simulink model "FOC_CHBI"  (R2025a)
settings: Solver=VariableStepAuto  StartTime=0.0  StopTime=6.5  RelTol=1e-3
InitFcn:
  | %% KHOI THONG SO DONG CO
  | U_nom=6000;%6600;           %dien ap dinh muc dong co
  | H=0.96;%0.9387;             %hieu suat dong co
  | Pn=1e6;%1750e3;         %Cong suat dinh muc dong co
  | cosphi=0.85;%0.9297;        %He so cong suat
  | Sn=Pn/cosphi;       %Cong suat toan phan
  | J=27.9;%34.8;                %Moment quan tinh
  | pc=2;%2;               %So cap cuc
  | fn=50;              %Tan so luoi
  | n=1490;%1486;             %Toc do dinh muc 2880
  | Mdm=6153;%(9.55*Pn*H)/n;  %Moment dinh muc
  | In=117;%Pn/(U_nom*H*cosphi*sqrt(3))   ;
  | Isd=sqrt(2)*In*sqrt(1-cosphi);
  | Isq=sqrt(2*In^2-Isd^2);
  | wrn=2*pi*(fn-(pc*n/60));               %Toc do truotdinh muc
  | Tr=Isq/(wrn*Isd) ;                   %Tinh 'Tr'trong cac cong thuc
  | %Xo=(sqrt(1-cosphi^2)-cosphi*Isd/Isq)*(Un*sqrt(2)/(sqrt(3)*In));
  | Xo=(sqrt(1-cosphi^2)-cosphi*Isd/Isq)*(U_nom/(sqrt(3)*In));
  | Xh=sqrt(2/3)*(U_nom/Isd) - Xo;
  | Rs=(wrn*Isd*Xh)/(2*pi*fn*Isq);
  | Rr=Rs;
  | o=Xo/Xh;
  | Ts=Xh/(2*pi*fn*Rs);
  | Tos=o*Ts;
  | Lr=Tr*Rr;
  | Lor=o*Lr;
  | Ls=Ts*Rs;
  | Los=o*Ls;
  | Lm=sqrt((1-o)*Ls*Lr);
  | %tham so dong co 2850e3Kw
  | %Rs=0.05;
  | %Rr = 0.062;
  | %Los = 0.957/(100*pi);
  | %Lor = 2.237/(100*pi);
  | %Lm = 34.826/(100*pi);
  | %Ts = (Lm +Los)/Rs;
  | %Tr = (Lm+Lor)/Rr;
  | %Lr = Lm + Lor;
  | %Ls = Lm + Los;
  | Udc = 1.1*6000/(0.612*12);%6600/(0.612*12);
  | Rt =18*Udc*Udc/1e6; %18*Udc*Udc/2010.6e3;
  | C_f = 5/(6*100*pi*Rt*0.001);
  | %Fan and Pumb Load Coeficient
  | TL0 = (2.0/100)*Mdm; %(2.0/100)*TN;
  | Omega_rated = n/9.55; %nN/9.55; %rad/s
  | LoadGain = (Mdm - TL0)/(Omega_rated*Omega_rated);
  | fs=5000;
  | %% THAM SO CAC BO DIEU KHIEN
  | %---------------- control volocity
  | epxilon = 0.7;
  | wn = 40;
  |      %P_w = (2*epxilon*wn*J)/pc;
  |     %I_w = wn*wn*J/pc;
  |  P_w = 60;%5;%15;%9;%12;%10;%(2*epxilon*wn*J)/pc
  |  I_w = 80;%150;%80;%100;%40;%50;%wn*wn*J/pc
  | %---------------- control current
  |     %P_id = Rs*Tos*fs/5;
  |     % I_id = Rs*Tos*fs/5/Tos;
  |      %P_iq = P_id;
  |      %I_iq = I_id;
  | ... (+9 lines)
StopFcn:
  | figure(1);
  | subplot(1,1,1); hold on; grid on;
  | plot(phi_ref.time, phi_ref.signals.values,'r--', 'Linewidth',1.5);
  | plot(phi.time, phi.signals.values,'b', 'Linewidth',1.5);
  | legend('phi*-rd','phi-rd');
  | title('Từ thông');
  | xlabel('Thời gian (s)'); ylabel('Wb');
  | 
  | 
  | figure(2);
  | subplot(2,1,1); hold on; grid on;
  | plot(torque.time, torque.signals.values,'r','Linewidth',1.5);
  | legend('Te');
  | title('Mô-men');
  | xlabel('Thời gian (s)'); ylabel('Nm');
  | 
  | subplot(2,1,2); hold on; grid on;
  | plot(speed_ref.time, speed_ref.signals.values,'r--','Linewidth',1.5);
  | plot(speed.time, speed.signals.values,'b','Linewidth',1.5);
  | legend('Tốc độ đặt','Tốc độ thực');
  | title('Tốc độ');
  | xlabel('Thời gian (s)'); ylabel('RPM');
  | 
  | figure(3)
  | 
  | subplot(2,1,1); hold on; grid on;
  | plot(isd_ref.time, isd_ref.signals.values,'r','Linewidth',1.5);
  | plot(isd.time, isd.signals.values,'b','Linewidth',1.5);
  | legend('isd*','isd');
  | title('Dòng điện isd');
  | xlabel('Thời gian (s)'); ylabel('A');
  | 
  | subplot(2,1,2); hold on; grid on;
  | plot(isq_ref.time, isq_ref.signals.values,'r','Linewidth',1.5);
  | plot(isq.time, isq.signals.values,'b','Linewidth',1.5);
  | legend('isq*','isq');
  | title('Dòng điện isq');
  | xlabel('Thời gian (s)'); ylabel('A');
  | 
  | figure(4)
  | 
  | subplot(2,1,1); hold on; grid on;
  | plot(va.time, va.signals.values,'b','Linewidth',1.5);
  | plot(vb.time, vb.signals.values,'k','Linewidth',1.5);
  | plot(vc.time, vc.signals.values,'r','Linewidth',1.5);
  | legend('Ua','Ub','Uc');
  | title('Điện áp pha');
  | xlabel('Thời gian (s)'); ylabel('V');
  | 
  | subplot(2,1,2); hold on; grid on;
  | plot(vab.time, vab.signals.values,'k','Linewidth',1.5);
  | plot(vbc.time, vbc.signals.values,'b','Linewidth',1.5);
  | plot(vca.time, vca.signals.values,'r','Linewidth',1.5);
  | legend('Uab','Ubc','Uca');
  | title('Điện áp dây');
  | xlabel('Thời gian (s)'); ylabel('V');
  | 
  | figure(5);
  | subplot(1,1,1); hold on; grid on;
  | plot(Ia.time, Ia.signals.values,'k','Linewidth',1.5);
  | ... (+5 lines)
undefined symbols (not defined in the file): sigbuilder_block
libraries: spsIGBTDiodeLib x72, spsTriangleGeneratorLib x36, spsSeriesRLCBranchLib x18, spsBreakerLib x18, spsUniversalBridgeLib x18, spsZigzagPhaseShiftingTransformerLib x15, spsVoltageMeasurementLib x8, spsACVoltageSourceLib x3, spsCurrentMeasurementLib x3, spsThreePhaseTransformerTwoWindingsLib x3, slpidlib x2, spsThreePhaseVIMeasurementLib x1
(part 2 of 3)

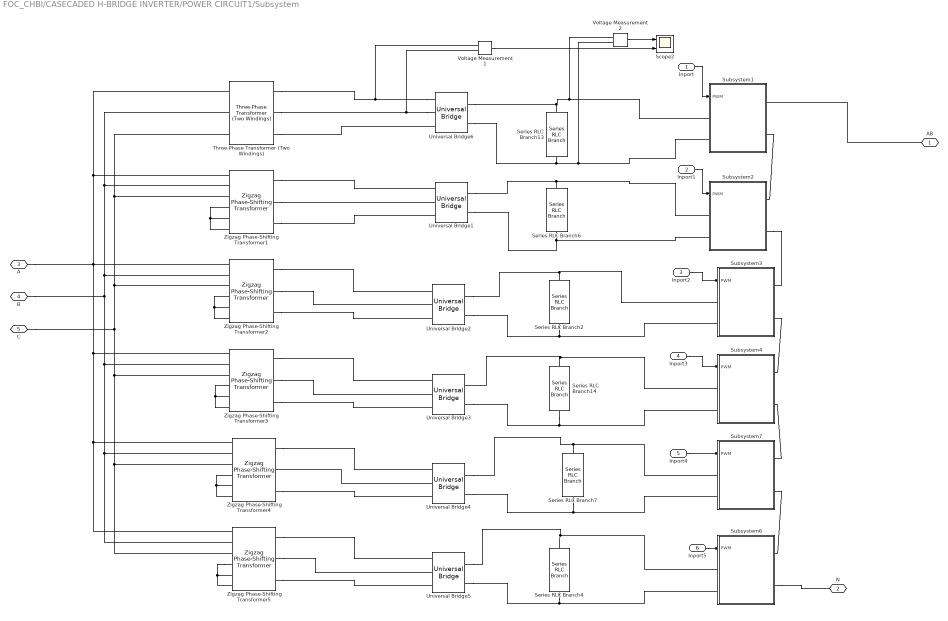
== system FOC_CHBI/CASECADED H-BRIDGE INVERTER/POWER CIRCUIT1/Subsystem ==
  Inport : Inport
  Inport1 : Inport  Port=2
  Inport2 : Inport  Port=3
  Inport3 : Inport  Port=4
  Inport4 : Inport  Port=5
  Inport5 : Inport  Port=6
  Scope2 : Scope  NumInputPorts=2
      settings: ActiveDisplayYMinimum=-1327.86919  ActiveDisplayYMaximum=1329.9135  DataLoggingVariableName=ScopeData6
  Series RLC Branch{2,4,6..7,13..14} (6 alike) : spsSeriesRLCBranchLib/Series RLC Branch  LConnTagsString=__new0  RConnTagsString=__new0  BranchType=C  Resistance=1  Inductance=1e-3  SetiL0=off  InitialCurrent=0  Capacitance=C_f  Setx0=off  InitialVoltage=0  Measurements=None
  Subsystem1 : Subsystem
  Subsystem2 : Subsystem
  Subsystem3 : Subsystem
  Subsystem4 : Subsystem
  Subsystem6 : Subsystem
  Subsystem7 : Subsystem
  Three-Phase Transformer (Two Windings) : spsThreePhaseTransformerTwoWindingsLib/Three-Phase Transformer (Two Windings)  Winding1Connection=Y  Winding2Connection=Y  CoreType=Three single-phase transformers  SetSaturation=off  Hysteresis=off  DataFile='hysteresis'  SetInitialFlux=off  Measurements=None  UNITS=SI  NominalPower=[ 100e6 , 50 ]  Winding1=[U_nom 0 0]  Winding2=[Udc/sqrt(2) 0 0]  Rm=66996  Lm=213.25  L0=0.5  Saturation=[0 0;1.6929 361.02;705.34 457.29]  InitialFluxes=[ 0.8 , -0.8 , 0.7 ]  BreakLoop=off  DiscreteSolver=Trapezoidal iterative  DataType=on  TransfoNumber=1
  Universal Bridge{1..6} (6 alike) : spsUniversalBridgeLib/Universal Bridge  Arms=3  SnubberResistance=1e5  SnubberCapacitance=inf  Device=Diodes  Ron=1e-3  Lon=0  ForwardVoltages="[  0  0  ]"  ForwardVoltage=0  GTOparameters=[ 10e-6 , 20e-6 ]  IGBTparameters=[ 1e-6 , 2e-6 ]  Measurements=None  Measurements_2=None  converterType=Rectifier
  Voltage Measurement1 : spsVoltageMeasurementLib/Voltage Measurement  PhasorSimulation=off  OutputType=Complex  PSBequivalent=0
  Voltage Measurement2 : spsVoltageMeasurementLib/Voltage Measurement  PhasorSimulation=off  OutputType=Complex  PSBequivalent=0
  Zigzag Phase-Shifting Transformer1 : spsZigzagPhaseShiftingTransformerLib/Zigzag Phase-Shifting Transformer  SecondaryConnection=Y  SetSaturation=off  SetInitialFlux=off  Measurements=None  UNITS=SI  NominalPower=[ 100e6 50]  PrimaryVoltage=U_nom  SecondaryVoltage="[ Udc/sqrt(2)  +10]"  Winding1=[0 0]  Winding2=[0 0]  Winding3=[0 0]  RmLm=[211.93 0.67458]  Rm=211.93  Saturation=[0 0;30.099 20.304;12541 25.719]  InitialFluxes=[0 0 0]  BreakLoop=off  DiscreteSolver=Trapezoidal iterative  DataType=on
      settings: LibrarySourceBlock=|
      | sps_lib/Power Grid Elements/Zigzag
      | Phase-Shifting Transformer
  Zigzag Phase-Shifting Transformer2 : spsZigzagPhaseShiftingTransformerLib/Zigzag Phase-Shifting Transformer  SecondaryConnection=Y  SetSaturation=off  SetInitialFlux=off  Measurements=None  UNITS=SI  NominalPower=[ 100e6 50]  PrimaryVoltage=U_nom  SecondaryVoltage="[Udc/sqrt(2)  +20]"  Winding1=[0 0]  Winding2=[0 0]  Winding3=[0 0]  RmLm=[232.76 0.74091]  Rm=232.76  Saturation=[0 0;28.721 21.279;11967 26.954]  InitialFluxes=[0 0 0]  BreakLoop=off  DiscreteSolver=Trapezoidal iterative  DataType=on
      settings: LibrarySourceBlock=|
      | sps_lib/Power Grid Elements/Zigzag
      | Phase-Shifting Transformer
  Zigzag Phase-Shifting Transformer3 : spsZigzagPhaseShiftingTransformerLib/Zigzag Phase-Shifting Transformer  SecondaryConnection=Y  SetSaturation=off  SetInitialFlux=off  Measurements=None  UNITS=SI  NominalPower=[ 100e6 50]  PrimaryVoltage=U_nom  SecondaryVoltage="[ Udc/sqrt(2)  +30]"  Winding1=[0 0]  Winding2=[0 0]  Winding3=[0 0]  RmLm=[240 0.76394]  Rm=240  Saturation=[0 0;28.284 21.608;11785 27.37]  InitialFluxes=[0 0 0]  BreakLoop=off  DiscreteSolver=Trapezoidal iterative  DataType=on
      settings: LibrarySourceBlock=|
      | sps_lib/Power Grid Elements/Zigzag
      | Phase-Shifting Transformer
  Zigzag Phase-Shifting Transformer4 : spsZigzagPhaseShiftingTransformerLib/Zigzag Phase-Shifting Transformer  SecondaryConnection=Y  SetSaturation=off  SetInitialFlux=off  Measurements=None  UNITS=SI  NominalPower=[ 100e6 50]  PrimaryVoltage=U_nom  SecondaryVoltage="[ Udc/sqrt(2)  +40]"  Winding1=[0 0]  Winding2=[0 0]  Winding3=[0 0]  RmLm=[232.76 0.74091]  Rm=232.76  Saturation=[0 0;28.721 21.279;11967 26.954]  InitialFluxes=[0 0 0]  BreakLoop=off  DiscreteSolver=Trapezoidal iterative  DataType=on
      settings: LibrarySourceBlock=|
      | sps_lib/Power Grid Elements/Zigzag
      | Phase-Shifting Transformer
  Zigzag Phase-Shifting Transformer5 : spsZigzagPhaseShiftingTransformerLib/Zigzag Phase-Shifting Transformer  SecondaryConnection=Y  SetSaturation=off  SetInitialFlux=off  Measurements=None  UNITS=SI  NominalPower=[ 100e6 50]  PrimaryVoltage=U_nom  SecondaryVoltage="[ Udc/sqrt(2)  +50]"  Winding1=[0 0]  Winding2=[0 0]  Winding3=[0 0]  RmLm=[211.93 0.67458]  Rm=211.93  Saturation=[0 0;30.099 20.304;12541 25.719]  InitialFluxes=[0 0 0]  BreakLoop=off  DiscreteSolver=Trapezoidal iterative  DataType=on
      settings: LibrarySourceBlock=|
      | sps_lib/Power Grid Elements/Zigzag
      | Phase-Shifting Transformer
  AB : PMIOPort  Side=Left
  N : PMIOPort  Port=2  Side=Left
  A : PMIOPort  Port=3  Side=Left
  B : PMIOPort  Port=4  Side=Left
  C : PMIOPort  Port=5  Side=Left
  wires:
  Voltage Measurement1/1 -> Scope2/2
  Voltage Measurement2/1 -> Scope2/1
  Inport5/1 -> Subsystem6/1(PWM)
  Inport4/1 -> Subsystem7/1(PWM)
  Inport3/1 -> Subsystem4/1(PWM)
  Inport2/1 -> Subsystem3/1(PWM)
  Inport1/1 -> Subsystem2/1(PWM)
  Inport/1 -> Subsystem1/1(PWM)
  connections:
  Universal Bridge3/RConn1 -- Subsystem4/LConn1 -- Series RLC Branch14/LConn1
  Universal Bridge5/RConn1 -- Subsystem6/LConn1 -- Series RLC Branch4/LConn1
  Universal Bridge4/RConn1 -- Subsystem7/LConn1 -- Series RLC Branch7/LConn1
  Universal Bridge1/RConn1 -- Subsystem2/LConn1 -- Series RLC Branch6/LConn1
  AB/RConn1 -- Subsystem1/RConn1
  Subsystem6/RConn2 -- N/RConn1
  Subsystem7/RConn2 -- Subsystem6/RConn1
  Subsystem7/RConn1 -- Subsystem4/RConn2
  Subsystem3/RConn2 -- Subsystem4/RConn1
  Subsystem2/RConn2 -- Subsystem3/RConn1
  Subsystem1/RConn2 -- Subsystem2/RConn1
  Universal Bridge6/LConn1 -- Voltage Measurement1/LConn1 -- Three-Phase Transformer (Two Windings)/RConn1
  Universal Bridge4/LConn2 -- Zigzag Phase-Shifting Transformer4/RConn2
  Zigzag Phase-Shifting Transformer4/RConn3 -- Universal Bridge4/LConn3
  Zigzag Phase-Shifting Transformer4/RConn1 -- Universal Bridge4/LConn1
  Zigzag Phase-Shifting Transformer2/LConn1 -- Zigzag Phase-Shifting Transformer3/LConn1 -- Zigzag Phase-Shifting Transformer4/LConn1 -- Zigzag Phase-Shifting Transformer5/LConn1 -- Zigzag Phase-Shifting Transformer1/LConn1 -- Three-Phase Transformer (Two Windings)/LConn1 -- A/RConn1
  Zigzag Phase-Shifting Transformer2/RConn2 -- Universal Bridge2/LConn2
  Zigzag Phase-Shifting Transformer3/RConn3 -- Universal Bridge3/LConn3
  Zigzag Phase-Shifting Transformer5/RConn3 -- Universal Bridge5/LConn3
  Zigzag Phase-Shifting Transformer2/RConn3 -- Universal Bridge2/LConn3
  Universal Bridge6/LConn2 -- Voltage Measurement1/LConn2 -- Three-Phase Transformer (Two Windings)/RConn2
  Zigzag Phase-Shifting Transformer3/RConn2 -- Universal Bridge3/LConn2
  Three-Phase Transformer (Two Windings)/RConn3 -- Universal Bridge6/LConn3
  Zigzag Phase-Shifting Transformer1/RConn1 -- Universal Bridge1/LConn1
  Zigzag Phase-Shifting Transformer1/LConn5 -- Zigzag Phase-Shifting Transformer1/LConn4 -- Zigzag Phase-Shifting Transformer1/LConn6
  Zigzag Phase-Shifting Transformer2/RConn1 -- Universal Bridge2/LConn1
  Zigzag Phase-Shifting Transformer2/LConn4 -- Zigzag Phase-Shifting Transformer2/LConn6 -- Zigzag Phase-Shifting Transformer2/LConn5
  Zigzag Phase-Shifting Transformer1/RConn2 -- Universal Bridge1/LConn2
  Universal Bridge6/RConn2 -- Series RLC Branch13/RConn1 -- Voltage Measurement2/LConn2 -- Subsystem1/LConn2
  B/RConn1 -- Zigzag Phase-Shifting Transformer2/LConn2 -- Three-Phase Transformer (Two Windings)/LConn2 -- Zigzag Phase-Shifting Transformer1/LConn2 -- Zigzag Phase-Shifting Transformer4/LConn2 -- Zigzag Phase-Shifting Transformer5/LConn2 -- Zigzag Phase-Shifting Transformer3/LConn2
  Zigzag Phase-Shifting Transformer5/LConn4 -- Zigzag Phase-Shifting Transformer5/LConn5 -- Zigzag Phase-Shifting Transformer5/LConn6
  Zigzag Phase-Shifting Transformer5/RConn1 -- Universal Bridge5/LConn1
  Universal Bridge5/RConn2 -- Subsystem6/LConn2 -- Series RLC Branch4/RConn1
  Universal Bridge3/RConn2 -- Series RLC Branch14/RConn1 -- Subsystem4/LConn2
  Zigzag Phase-Shifting Transformer4/LConn5 -- Zigzag Phase-Shifting Transformer4/LConn4 -- Zigzag Phase-Shifting Transformer4/LConn6
  Series RLC Branch6/RConn1 -- Universal Bridge1/RConn2 -- Subsystem2/LConn2
  Universal Bridge2/RConn1 -- Subsystem3/LConn1 -- Series RLC Branch2/LConn1
  Zigzag Phase-Shifting Transformer1/RConn3 -- Universal Bridge1/LConn3
  Zigzag Phase-Shifting Transformer5/LConn3 -- Zigzag Phase-Shifting Transformer3/LConn3 -- C/RConn1 -- Zigzag Phase-Shifting Transformer2/LConn3 -- Zigzag Phase-Shifting Transformer1/LConn3 -- Three-Phase Transformer (Two Windings)/LConn3 -- Zigzag Phase-Shifting Transformer4/LConn3
  Universal Bridge4/RConn2 -- Subsystem7/LConn2 -- Series RLC Branch7/RConn1
  Universal Bridge2/RConn2 -- Series RLC Branch2/RConn1 -- Subsystem3/LConn2
  Universal Bridge6/RConn1 -- Subsystem1/LConn1 -- Voltage Measurement2/LConn1 -- Series RLC Branch13/LConn1
  Zigzag Phase-Shifting Transformer3/LConn4 -- Zigzag Phase-Shifting Transformer3/LConn6 -- Zigzag Phase-Shifting Transformer3/LConn5
  Zigzag Phase-Shifting Transformer3/RConn1 -- Universal Bridge3/LConn1
  Zigzag Phase-Shifting Transformer5/RConn2 -- Universal Bridge5/LConn2

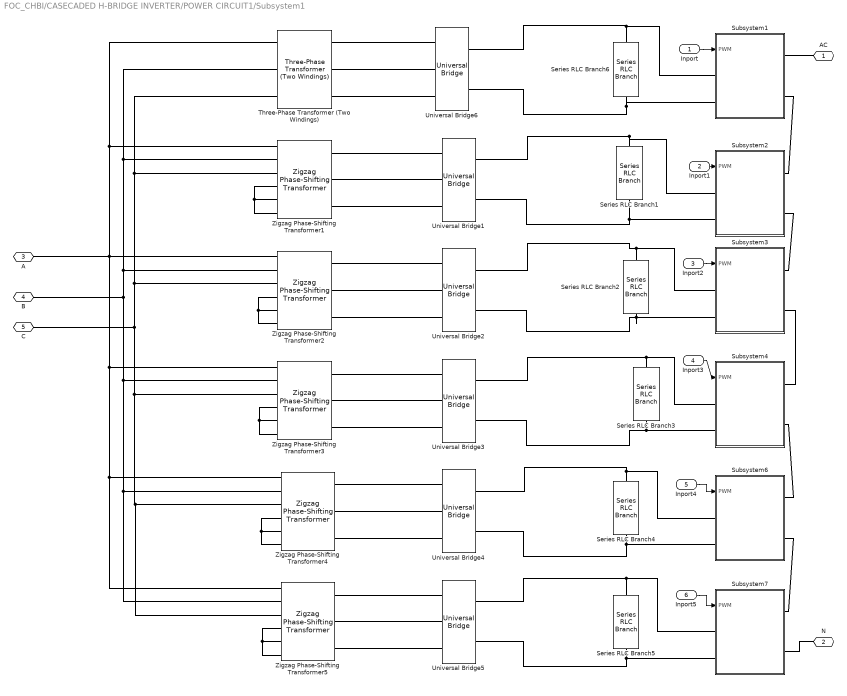
== system FOC_CHBI/CASECADED H-BRIDGE INVERTER/POWER CIRCUIT1/Subsystem1 ==
  Inport : Inport
  Inport1 : Inport  Port=2
  Inport2 : Inport  Port=3
  Inport3 : Inport  Port=4
  Inport4 : Inport  Port=5
  Inport5 : Inport  Port=6
  Series RLC Branch{1..6} (6 alike) : spsSeriesRLCBranchLib/Series RLC Branch  LConnTagsString=__new0  RConnTagsString=__new0  BranchType=C  Resistance=1  Inductance=1e-3  SetiL0=off  InitialCurrent=0  Capacitance=C_f  Setx0=off  InitialVoltage=0  Measurements=None
  Subsystem1 : Subsystem
  Subsystem2 : Subsystem
  Subsystem3 : Subsystem
  Subsystem4 : Subsystem
  Subsystem6 : Subsystem
  Subsystem7 : Subsystem
  Three-Phase Transformer (Two Windings) : spsThreePhaseTransformerTwoWindingsLib/Three-Phase Transformer (Two Windings)  Winding1Connection=Y  Winding2Connection=Y  CoreType=Three single-phase transformers  SetSaturation=off  Hysteresis=off  DataFile='hysteresis'  SetInitialFlux=off  Measurements=None  UNITS=SI  NominalPower=[ 100e6 , 50 ]  Winding1=[U_nom 0 0]  Winding2=[Udc/sqrt(2) 0 0]  Rm=66996  Lm=213.25  L0=0.5  Saturation=[0 0;1.6929 361.02;705.34 457.29]  InitialFluxes=[ 0.8 , -0.8 , 0.7 ]  BreakLoop=off  DiscreteSolver=Trapezoidal iterative  DataType=on  TransfoNumber=1
  Universal Bridge{1..6} (6 alike) : spsUniversalBridgeLib/Universal Bridge  Arms=3  SnubberResistance=1e5  SnubberCapacitance=inf  Device=Diodes  Ron=1e-3  Lon=0  ForwardVoltages="[  0  0  ]"  ForwardVoltage=0  GTOparameters=[ 10e-6 , 20e-6 ]  IGBTparameters=[ 1e-6 , 2e-6 ]  Measurements=None  Measurements_2=None  converterType=Rectifier
  Zigzag Phase-Shifting Transformer1 : spsZigzagPhaseShiftingTransformerLib/Zigzag Phase-Shifting Transformer  SecondaryConnection=Y  SetSaturation=off  SetInitialFlux=off  Measurements=None  UNITS=SI  NominalPower=[ 100e6 50]  PrimaryVoltage=U_nom  SecondaryVoltage=[ Udc/sqrt(2) +10]  Winding1=[0 0]  Winding2=[0 0]  Winding3=[0 0]  RmLm=[211.93 0.67458]  Rm=211.93  Saturation=[0 0;30.099 20.304;12541 25.719]  InitialFluxes=[0 0 0]  BreakLoop=off  DiscreteSolver=Trapezoidal iterative  DataType=on
      settings: LibrarySourceBlock=|
      | sps_lib/Power Grid Elements/Zigzag
      | Phase-Shifting Transformer
  Zigzag Phase-Shifting Transformer2 : spsZigzagPhaseShiftingTransformerLib/Zigzag Phase-Shifting Transformer  SecondaryConnection=Y  SetSaturation=off  SetInitialFlux=off  Measurements=None  UNITS=SI  NominalPower=[ 100e6 50]  PrimaryVoltage=U_nom  SecondaryVoltage="[ Udc/sqrt(2)  +20]"  Winding1=[0 0]  Winding2=[0 0]  Winding3=[0 0]  RmLm=[232.76 0.74091]  Rm=232.76  Saturation=[0 0;28.721 21.279;11967 26.954]  InitialFluxes=[0 0 0]  BreakLoop=off  DiscreteSolver=Trapezoidal iterative  DataType=on
      settings: LibrarySourceBlock=|
      | sps_lib/Power Grid Elements/Zigzag
      | Phase-Shifting Transformer
  Zigzag Phase-Shifting Transformer3 : spsZigzagPhaseShiftingTransformerLib/Zigzag Phase-Shifting Transformer  SecondaryConnection=Y  SetSaturation=off  SetInitialFlux=off  Measurements=None  UNITS=SI  NominalPower=[ 100e6 50]  PrimaryVoltage=U_nom  SecondaryVoltage=[ Udc/sqrt(2) +30]  Winding1=[0 0]  Winding2=[0 0]  Winding3=[0 0]  RmLm=[240 0.76394]  Rm=240  Saturation=[0 0;28.284 21.608;11785 27.37]  InitialFluxes=[0 0 0]  BreakLoop=off  DiscreteSolver=Trapezoidal iterative  DataType=on
      settings: LibrarySourceBlock=|
      | sps_lib/Power Grid Elements/Zigzag
      | Phase-Shifting Transformer
  Zigzag Phase-Shifting Transformer4 : spsZigzagPhaseShiftingTransformerLib/Zigzag Phase-Shifting Transformer  SecondaryConnection=Y  SetSaturation=off  SetInitialFlux=off  Measurements=None  UNITS=SI  NominalPower=[ 100e6 50]  PrimaryVoltage=U_nom  SecondaryVoltage="[ Udc/sqrt(2)  +40]"  Winding1=[0 0]  Winding2=[0 0]  Winding3=[0 0]  RmLm=[232.76 0.74091]  Rm=232.76  Saturation=[0 0;28.721 21.279;11967 26.954]  InitialFluxes=[0 0 0]  BreakLoop=off  DiscreteSolver=Trapezoidal iterative  DataType=on
      settings: LibrarySourceBlock=|
      | sps_lib/Power Grid Elements/Zigzag
      | Phase-Shifting Transformer
  Zigzag Phase-Shifting Transformer5 : spsZigzagPhaseShiftingTransformerLib/Zigzag Phase-Shifting Transformer  SecondaryConnection=Y  SetSaturation=off  SetInitialFlux=off  Measurements=None  UNITS=SI  NominalPower=[ 100e6 50]  PrimaryVoltage=U_nom  SecondaryVoltage="[ Udc/sqrt(2)  +50]"  Winding1=[0 0]  Winding2=[0 0]  Winding3=[0 0]  RmLm=[211.93 0.67458]  Rm=211.93  Saturation=[0 0;30.099 20.304;12541 25.719]  InitialFluxes=[0 0 0]  BreakLoop=off  DiscreteSolver=Trapezoidal iterative  DataType=on
      settings: LibrarySourceBlock=|
      | sps_lib/Power Grid Elements/Zigzag
      | Phase-Shifting Transformer
  AC : PMIOPort  Side=Left
  N : PMIOPort  Port=2  Side=Left
  A : PMIOPort  Port=3  Side=Left
  B : PMIOPort  Port=4  Side=Left
  C : PMIOPort  Port=5  Side=Left
  wires:
  Inport5/1 -> Subsystem7/1(PWM)
  Inport4/1 -> Subsystem6/1(PWM)
  Inport3/1 -> Subsystem4/1(PWM)
  Inport2/1 -> Subsystem3/1(PWM)
  Inport1/1 -> Subsystem2/1(PWM)
  Inport/1 -> Subsystem1/1(PWM)
  connections:
  Universal Bridge5/RConn1 -- Subsystem7/LConn1 -- Series RLC Branch5/LConn1
  Universal Bridge6/RConn1 -- Series RLC Branch6/LConn1 -- Subsystem1/LConn1
  Universal Bridge4/RConn1 -- Subsystem6/LConn1 -- Series RLC Branch4/LConn1
  Universal Bridge3/RConn1 -- Series RLC Branch3/LConn1 -- Subsystem4/LConn1
  Universal Bridge2/RConn1 -- Series RLC Branch2/LConn1 -- Subsystem3/LConn1
  Universal Bridge1/RConn1 -- Series RLC Branch1/LConn1 -- Subsystem2/LConn1
  Universal Bridge5/RConn2 -- Subsystem7/LConn2 -- Series RLC Branch5/RConn1
  Series RLC Branch4/RConn1 -- Subsystem6/LConn2 -- Universal Bridge4/RConn2
  Subsystem4/LConn2 -- Series RLC Branch3/RConn1 -- Universal Bridge3/RConn2
  Universal Bridge2/RConn2 -- Series RLC Branch2/RConn1 -- Subsystem3/LConn2
  Subsystem2/LConn2 -- Series RLC Branch1/RConn1 -- Universal Bridge1/RConn2
  Universal Bridge6/RConn2 -- Series RLC Branch6/RConn1 -- Subsystem1/LConn2
  Universal Bridge3/LConn1 -- Zigzag Phase-Shifting Transformer3/RConn1
  Universal Bridge3/LConn2 -- Zigzag Phase-Shifting Transformer3/RConn2
  Universal Bridge3/LConn3 -- Zigzag Phase-Shifting Transformer3/RConn3
  Universal Bridge4/LConn1 -- Zigzag Phase-Shifting Transformer4/RConn1
  Universal Bridge4/LConn2 -- Zigzag Phase-Shifting Transformer4/RConn2
  Universal Bridge4/LConn3 -- Zigzag Phase-Shifting Transformer4/RConn3
  Universal Bridge5/LConn3 -- Zigzag Phase-Shifting Transformer5/RConn3
  Universal Bridge5/LConn2 -- Zigzag Phase-Shifting Transformer5/RConn2
  Universal Bridge5/LConn1 -- Zigzag Phase-Shifting Transformer5/RConn1
  Universal Bridge6/LConn3 -- Three-Phase Transformer (Two Windings)/RConn3
  Universal Bridge6/LConn1 -- Three-Phase Transformer (Two Windings)/RConn1
  Universal Bridge6/LConn2 -- Three-Phase Transformer (Two Windings)/RConn2
  Universal Bridge1/LConn3 -- Zigzag Phase-Shifting Transformer1/RConn3
  Universal Bridge1/LConn2 -- Zigzag Phase-Shifting Transformer1/RConn2
  Universal Bridge1/LConn1 -- Zigzag Phase-Shifting Transformer1/RConn1
  AC/RConn1 -- Subsystem1/RConn1
  Subsystem7/RConn2 -- N/RConn1
  Subsystem6/RConn2 -- Subsystem7/RConn1
  Subsystem6/RConn1 -- Subsystem4/RConn2
  Subsystem3/RConn2 -- Subsystem4/RConn1
  Subsystem2/RConn2 -- Subsystem3/RConn1
  Subsystem1/RConn2 -- Subsystem2/RConn1
  Zigzag Phase-Shifting Transformer2/LConn1 -- Zigzag Phase-Shifting Transformer3/LConn1 -- Zigzag Phase-Shifting Transformer4/LConn1 -- Zigzag Phase-Shifting Transformer5/LConn1 -- Zigzag Phase-Shifting Transformer1/LConn1 -- Three-Phase Transformer (Two Windings)/LConn1 -- A/RConn1
  Zigzag Phase-Shifting Transformer2/RConn2 -- Universal Bridge2/LConn2
  Zigzag Phase-Shifting Transformer2/RConn3 -- Universal Bridge2/LConn3
  Zigzag Phase-Shifting Transformer1/LConn6 -- Zigzag Phase-Shifting Transformer1/LConn5 -- Zigzag Phase-Shifting Transformer1/LConn4
  Zigzag Phase-Shifting Transformer2/RConn1 -- Universal Bridge2/LConn1
  Zigzag Phase-Shifting Transformer2/LConn5 -- Zigzag Phase-Shifting Transformer2/LConn4 -- Zigzag Phase-Shifting Transformer2/LConn6
  Zigzag Phase-Shifting Transformer2/LConn2 -- B/RConn1 -- Zigzag Phase-Shifting Transformer3/LConn2 -- Zigzag Phase-Shifting Transformer4/LConn2 -- Zigzag Phase-Shifting Transformer5/LConn2 -- Three-Phase Transformer (Two Windings)/LConn2 -- Zigzag Phase-Shifting Transformer1/LConn2
  Zigzag Phase-Shifting Transformer5/LConn4 -- Zigzag Phase-Shifting Transformer5/LConn6 -- Zigzag Phase-Shifting Transformer5/LConn5
  Zigzag Phase-Shifting Transformer4/LConn5 -- Zigzag Phase-Shifting Transformer4/LConn6 -- Zigzag Phase-Shifting Transformer4/LConn4
  Zigzag Phase-Shifting Transformer1/LConn3 -- Three-Phase Transformer (Two Windings)/LConn3 -- Zigzag Phase-Shifting Transformer2/LConn3 -- C/RConn1 -- Zigzag Phase-Shifting Transformer4/LConn3 -- Zigzag Phase-Shifting Transformer5/LConn3 -- Zigzag Phase-Shifting Transformer3/LConn3
  Zigzag Phase-Shifting Transformer3/LConn5 -- Zigzag Phase-Shifting Transformer3/LConn4 -- Zigzag Phase-Shifting Transformer3/LConn6

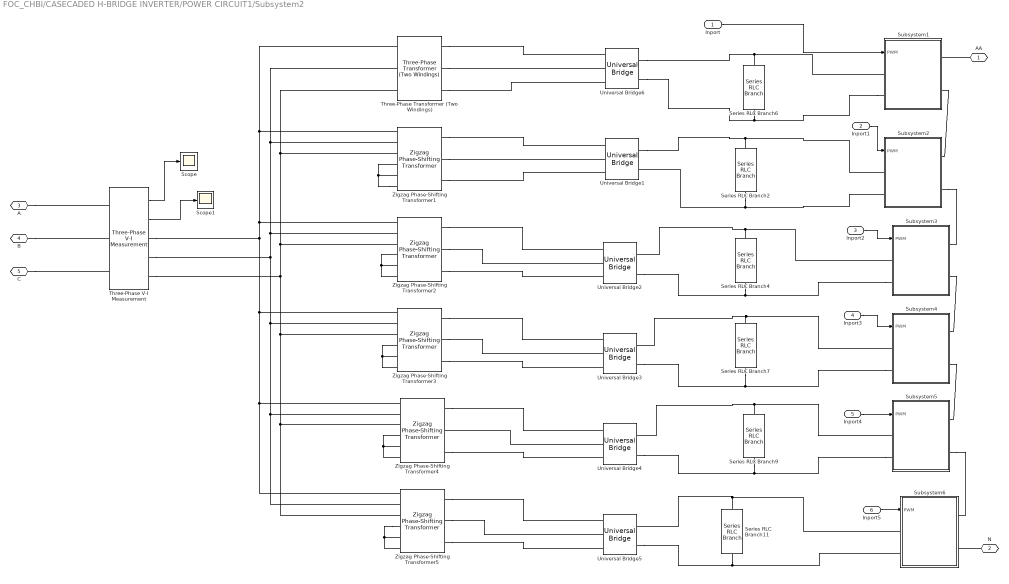
== system FOC_CHBI/CASECADED H-BRIDGE INVERTER/POWER CIRCUIT1/Subsystem2 ==
  Inport : Inport
  Inport1 : Inport  Port=2
  Inport2 : Inport  Port=3
  Inport3 : Inport  Port=4
  Inport4 : Inport  Port=5
  Inport5 : Inport  Port=6
  Scope : Scope
      settings: ActiveDisplayYMinimum=-10606.60172  ActiveDisplayYMaximum=10606.60172
  Scope1 : Scope
      settings: ActiveDisplayYMinimum=-356805.10971  ActiveDisplayYMaximum=356941.26542  DataLoggingVariableName=ScopeData2
  Series RLC Branch{2,4,6..7,9,11} (6 alike) : spsSeriesRLCBranchLib/Series RLC Branch  LConnTagsString=__new0  RConnTagsString=__new0  BranchType=C  Resistance=1  Inductance=1e-3  SetiL0=off  InitialCurrent=0  Capacitance=C_f  Setx0=off  InitialVoltage=0  Measurements=None
  Subsystem1 : Subsystem
  Subsystem2 : Subsystem
  Subsystem3 : Subsystem
  Subsystem4 : Subsystem
  Subsystem5 : Subsystem
  Subsystem6 : Subsystem
  Three-Phase Transformer (Two Windings) : spsThreePhaseTransformerTwoWindingsLib/Three-Phase Transformer (Two Windings)  Winding1Connection=Y  Winding2Connection=Y  CoreType=Three single-phase transformers  SetSaturation=off  Hysteresis=off  DataFile='hysteresis'  SetInitialFlux=off  Measurements=None  UNITS=SI  NominalPower=[ 100e6 , 50 ]  Winding1=[U_nom 0 0]  Winding2=[Udc/sqrt(2) 0 0]  Rm=66996  Lm=213.25  L0=0.5  Saturation=[0 0;1.6929 361.02;705.34 457.29]  InitialFluxes=[ 0.8 , -0.8 , 0.7 ]  BreakLoop=off  DiscreteSolver=Trapezoidal iterative  DataType=on  TransfoNumber=1
  Three-Phase V-I Measurement : spsThreePhaseVIMeasurementLib/Three-Phase V-I Measurement  VoltageMeasurement=phase-to-phase  SetLabelV=off  LabelV=Vabc  Vpu=off  VpuLL=off  CurrentMeasurement=yes  SetLabelI=off  LabelI=Iabc  Ipu=off  Pbase=100e6  Vbase=500e3  OutputType=Complex  PhasorSimulation=off  PSBequivalent=0
  Universal Bridge{1..6} (6 alike) : spsUniversalBridgeLib/Universal Bridge  Arms=3  SnubberResistance=1e5  SnubberCapacitance=inf  Device=Diodes  Ron=1e-3  Lon=0  ForwardVoltages="[  0  0  ]"  ForwardVoltage=0  GTOparameters=[ 10e-6 , 20e-6 ]  IGBTparameters=[ 1e-6 , 2e-6 ]  Measurements=None  Measurements_2=None  converterType=Rectifier
  Zigzag Phase-Shifting Transformer1 : spsZigzagPhaseShiftingTransformerLib/Zigzag Phase-Shifting Transformer  SecondaryConnection=Y  SetSaturation=off  SetInitialFlux=off  Measurements=None  UNITS=SI  NominalPower=[ 100e6 50]  PrimaryVoltage=U_nom  SecondaryVoltage=[Udc/sqrt(2) +10]  Winding1=[0 0]  Winding2=[0 0]  Winding3=[0 0]  RmLm=[211.93 0.67458]  Rm=211.93  Saturation=[0 0;30.099 20.304;12541 25.719]  InitialFluxes=[0 0 0]  BreakLoop=off  DiscreteSolver=Trapezoidal iterative  DataType=on
      settings: LibrarySourceBlock=|
      | sps_lib/Power Grid Elements/Zigzag
      | Phase-Shifting Transformer
  Zigzag Phase-Shifting Transformer2 : spsZigzagPhaseShiftingTransformerLib/Zigzag Phase-Shifting Transformer  SecondaryConnection=Y  SetSaturation=off  SetInitialFlux=off  Measurements=None  UNITS=SI  NominalPower=[ 100e6 50]  PrimaryVoltage=U_nom  SecondaryVoltage="[Udc/sqrt(2)  +20]"  Winding1=[0 0]  Winding2=[0 0]  Winding3=[0 0]  RmLm=[232.76 0.74091]  Rm=232.76  Saturation=[0 0;28.721 21.279;11967 26.954]  InitialFluxes=[0 0 0]  BreakLoop=off  DiscreteSolver=Trapezoidal iterative  DataType=on
      settings: LibrarySourceBlock=|
      | sps_lib/Power Grid Elements/Zigzag
      | Phase-Shifting Transformer
  Zigzag Phase-Shifting Transformer3 : spsZigzagPhaseShiftingTransformerLib/Zigzag Phase-Shifting Transformer  SecondaryConnection=Y  SetSaturation=off  SetInitialFlux=off  Measurements=None  UNITS=SI  NominalPower=[ 100e6 50]  PrimaryVoltage=U_nom  SecondaryVoltage="[Udc/sqrt(2)  +30]"  Winding1=[0 0]  Winding2=[0 0]  Winding3=[0 0]  RmLm=[240 0.76394]  Rm=240  Saturation=[0 0;28.284 21.608;11785 27.37]  InitialFluxes=[0 0 0]  BreakLoop=off  DiscreteSolver=Trapezoidal iterative  DataType=on
      settings: LibrarySourceBlock=|
      | sps_lib/Power Grid Elements/Zigzag
      | Phase-Shifting Transformer
  Zigzag Phase-Shifting Transformer4 : spsZigzagPhaseShiftingTransformerLib/Zigzag Phase-Shifting Transformer  SecondaryConnection=Y  SetSaturation=off  SetInitialFlux=off  Measurements=None  UNITS=SI  NominalPower=[ 100e6 50]  PrimaryVoltage=U_nom  SecondaryVoltage="[ Udc/sqrt(2)  +40]"  Winding1=[0 0]  Winding2=[0 0]  Winding3=[0 0]  RmLm=[232.76 0.74091]  Rm=232.76  Saturation=[0 0;28.721 21.279;11967 26.954]  InitialFluxes=[0 0 0]  BreakLoop=off  DiscreteSolver=Trapezoidal iterative  DataType=on
      settings: LibrarySourceBlock=|
      | sps_lib/Power Grid Elements/Zigzag
      | Phase-Shifting Transformer
  Zigzag Phase-Shifting Transformer5 : spsZigzagPhaseShiftingTransformerLib/Zigzag Phase-Shifting Transformer  SecondaryConnection=Y  SetSaturation=off  SetInitialFlux=off  Measurements=None  UNITS=SI  NominalPower=[ 100e6 50]  PrimaryVoltage=U_nom  SecondaryVoltage="[ Udc/sqrt(2)  +50]"  Winding1=[0 0]  Winding2=[0 0]  Winding3=[0 0]  RmLm=[211.93 0.67458]  Rm=211.93  Saturation=[0 0;30.099 20.304;12541 25.719]  InitialFluxes=[0 0 0]  BreakLoop=off  DiscreteSolver=Trapezoidal iterative  DataType=on
      settings: LibrarySourceBlock=|
      | sps_lib/Power Grid Elements/Zigzag
      | Phase-Shifting Transformer
  AA : PMIOPort  Side=Left
  N : PMIOPort  Port=2  Side=Left
  A : PMIOPort  Port=3  Side=Left
  B : PMIOPort  Port=4  Side=Left
  C : PMIOPort  Port=5  Side=Left
  wires:
  Inport/1 -> Subsystem1/1(PWM)
  Inport5/1 -> Subsystem6/1(PWM)
  Inport4/1 -> Subsystem5/1(PWM)
  Inport3/1 -> Subsystem4/1(PWM)
  Inport2/1 -> Subsystem3/1(PWM)
  Inport1/1 -> Subsystem2/1(PWM)
  Three-Phase V-I Measurement/1 -> Scope/1
  Three-Phase V-I Measurement/2 -> Scope1/1
  connections:
  C/RConn1 -- Three-Phase V-I Measurement/LConn3
  B/RConn1 -- Three-Phase V-I Measurement/LConn2
  A/RConn1 -- Three-Phase V-I Measurement/LConn1
  Universal Bridge5/RConn1 -- Subsystem6/LConn1 -- Series RLC Branch11/LConn1
  Universal Bridge4/RConn1 -- Subsystem5/LConn1 -- Series RLC Branch9/LConn1
  Universal Bridge3/RConn1 -- Subsystem4/LConn1 -- Series RLC Branch7/LConn1
  Universal Bridge2/RConn1 -- Series RLC Branch4/LConn1 -- Subsystem3/LConn1
  N/RConn1 -- Subsystem6/RConn2
  AA/RConn1 -- Subsystem1/RConn1
  Subsystem5/RConn2 -- Subsystem6/RConn1
  Subsystem4/RConn2 -- Subsystem5/RConn1
  Subsystem3/RConn2 -- Subsystem4/RConn1
  Subsystem2/RConn2 -- Subsystem3/RConn1
  Subsystem1/RConn2 -- Subsystem2/RConn1
  Three-Phase Transformer (Two Windings)/RConn1 -- Universal Bridge6/LConn1
  Universal Bridge4/LConn2 -- Zigzag Phase-Shifting Transformer4/RConn2
  Zigzag Phase-Shifting Transformer4/RConn3 -- Universal Bridge4/LConn3
  Zigzag Phase-Shifting Transformer4/RConn1 -- Universal Bridge4/LConn1
  Zigzag Phase-Shifting Transformer2/RConn2 -- Universal Bridge2/LConn2
  Zigzag Phase-Shifting Transformer3/RConn3 -- Universal Bridge3/LConn3
  Zigzag Phase-Shifting Transformer5/RConn3 -- Universal Bridge5/LConn3
  Zigzag Phase-Shifting Transformer2/RConn3 -- Universal Bridge2/LConn3
  Three-Phase Transformer (Two Windings)/RConn2 -- Universal Bridge6/LConn2
  Zigzag Phase-Shifting Transformer3/RConn2 -- Universal Bridge3/LConn2
  Three-Phase Transformer (Two Windings)/RConn3 -- Universal Bridge6/LConn3
  Zigzag Phase-Shifting Transformer1/RConn1 -- Universal Bridge1/LConn1
  Zigzag Phase-Shifting Transformer1/LConn6 -- Zigzag Phase-Shifting Transformer1/LConn5 -- Zigzag Phase-Shifting Transformer1/LConn4
  Zigzag Phase-Shifting Transformer2/RConn1 -- Universal Bridge2/LConn1
  Zigzag Phase-Shifting Transformer2/LConn5 -- Zigzag Phase-Shifting Transformer2/LConn4 -- Zigzag Phase-Shifting Transformer2/LConn6
  Zigzag Phase-Shifting Transformer1/RConn2 -- Universal Bridge1/LConn2
  Subsystem1/LConn2 -- Series RLC Branch6/RConn1 -- Universal Bridge6/RConn2
  Three-Phase V-I Measurement/RConn2 -- Zigzag Phase-Shifting Transformer3/LConn2 -- Zigzag Phase-Shifting Transformer4/LConn2 -- Zigzag Phase-Shifting Transformer5/LConn2 -- Zigzag Phase-Shifting Transformer2/LConn2 -- Three-Phase Transformer (Two Windings)/LConn2 -- Zigzag Phase-Shifting Transformer1/LConn2
  Zigzag Phase-Shifting Transformer5/LConn4 -- Zigzag Phase-Shifting Transformer5/LConn6 -- Zigzag Phase-Shifting Transformer5/LConn5
  Zigzag Phase-Shifting Transformer5/RConn1 -- Universal Bridge5/LConn1
  Series RLC Branch11/RConn1 -- Subsystem6/LConn2 -- Universal Bridge5/RConn2
  Subsystem4/LConn2 -- Series RLC Branch7/RConn1 -- Universal Bridge3/RConn2
  Zigzag Phase-Shifting Transformer4/LConn5 -- Zigzag Phase-Shifting Transformer4/LConn6 -- Zigzag Phase-Shifting Transformer4/LConn4
  Universal Bridge1/RConn2 -- Series RLC Branch2/RConn1 -- Subsystem2/LConn2
  Universal Bridge1/RConn1 -- Series RLC Branch2/LConn1 -- Subsystem2/LConn1
  Zigzag Phase-Shifting Transformer1/RConn3 -- Universal Bridge1/LConn3
  Zigzag Phase-Shifting Transformer4/LConn3 -- Zigzag Phase-Shifting Transformer5/LConn3 -- Zigzag Phase-Shifting Transformer3/LConn3 -- Zigzag Phase-Shifting Transformer2/LConn3 -- Zigzag Phase-Shifting Transformer1/LConn3 -- Three-Phase Transformer (Two Windings)/LConn3 -- Three-Phase V-I Measurement/RConn3
  Subsystem5/LConn2 -- Series RLC Branch9/RConn1 -- Universal Bridge4/RConn2
  Subsystem3/LConn2 -- Series RLC Branch4/RConn1 -- Universal Bridge2/RConn2
  Universal Bridge6/RConn1 -- Series RLC Branch6/LConn1 -- Subsystem1/LConn1
  Zigzag Phase-Shifting Transformer3/LConn5 -- Zigzag Phase-Shifting Transformer3/LConn4 -- Zigzag Phase-Shifting Transformer3/LConn6
  Zigzag Phase-Shifting Transformer2/LConn1 -- Zigzag Phase-Shifting Transformer1/LConn1 -- Three-Phase Transformer (Two Windings)/LConn1 -- Three-Phase V-I Measurement/RConn1 -- Zigzag Phase-Shifting Transformer3/LConn1 -- Zigzag Phase-Shifting Transformer4/LConn1 -- Zigzag Phase-Shifting Transformer5/LConn1
  Zigzag Phase-Shifting Transformer3/RConn1 -- Universal Bridge3/LConn1
  Zigzag Phase-Shifting Transformer5/RConn2 -- Universal Bridge5/LConn2

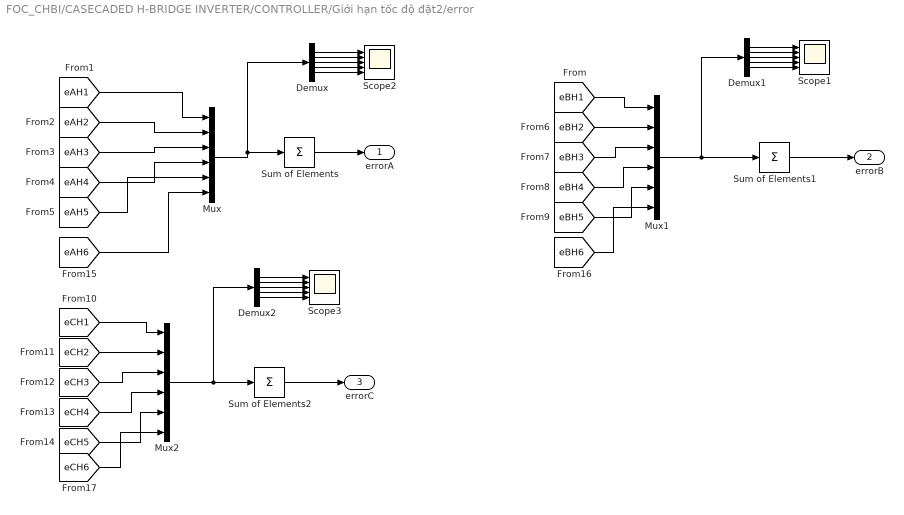
== system FOC_CHBI/CASECADED H-BRIDGE INVERTER/CONTROLLER/Giới hạn tốc độ đặt2/error ==
  Demux : Demux  Outputs=5
  Demux1 : Demux  Outputs=5
  Demux2 : Demux  Outputs=5
  Mux : Mux  Inputs=6
  Mux1 : Mux  Inputs=6
  Mux2 : Mux  Inputs=6
  Scope1 : Scope  NumInputPorts=5
      settings: ActiveDisplayYMinimum=-1  ActiveDisplayYMaximum=1
  Scope2 : Scope  NumInputPorts=5
      settings: ActiveDisplayYMinimum=-1  ActiveDisplayYMaximum=1  DataLoggingVariableName=ScopeData3
  Scope3 : Scope  NumInputPorts=5
      settings: ActiveDisplayYMinimum=-1  ActiveDisplayYMaximum=1  DataLoggingVariableName=ScopeData2
  Sum of Elements : Sum  Inputs=+
  Sum of Elements1 : Sum  Inputs=+
  Sum of Elements2 : Sum  Inputs=+
  errorA : Outport  VectorParamsAs1DForOutWhenUnconnected=off
  errorB : Outport  Port=2  VectorParamsAs1DForOutWhenUnconnected=off
  errorC : Outport  Port=3  VectorParamsAs1DForOutWhenUnconnected=off
  wires:
  [eCH6] -> Mux2/6
  [eBH6] -> Mux1/6
  [eAH6] -> Mux/6
  [eAH5] -> Mux/5
  [eAH4] -> Mux/4
  [eAH2] -> Mux/2
  [eAH3] -> Mux/3
  Mux/1 -> Sum of Elements/1, Demux/1
  Demux/3 -> Scope2/3
  Demux/2 -> Scope2/2
  Demux/1 -> Scope2/1
  Demux/4 -> Scope2/4
  Demux/5 -> Scope2/5
  Demux1/5 -> Scope1/5
  Demux1/4 -> Scope1/4
  Demux1/1 -> Scope1/1
  Demux1/2 -> Scope1/2
  Demux1/3 -> Scope1/3
  Mux1/1 -> Sum of Elements1/1, Demux1/1
  Mux2/1 -> Sum of Elements2/1, Demux2/1
  Demux2/3 -> Scope3/3
  Demux2/2 -> Scope3/2
  Demux2/1 -> Scope3/1
  Demux2/4 -> Scope3/4
  Demux2/5 -> Scope3/5
  Sum of Elements/1 -> errorA/1
  Sum of Elements1/1 -> errorB/1
  Sum of Elements2/1 -> errorC/1
  [eAH1] -> Mux/1
  [eBH2] -> Mux1/2
  [eBH3] -> Mux1/3
  [eBH4] -> Mux1/4
  [eBH5] -> Mux1/5
  [eBH1] -> Mux1/1
  [eCH2] -> Mux2/2
  [eCH5] -> Mux2/5
  [eCH3] -> Mux2/3
  [eCH1] -> Mux2/1
  [eCH4] -> Mux2/4

== system FOC_CHBI/CASECADED H-BRIDGE INVERTER/CONTROLLER/R_i1/id ==
  In2 : Inport
  Constant : Constant  Value=T  SampleTime=T
  Constant1 : Constant  Value=Kp  SampleTime=T
  Constant2 : Constant  Value=Ki  SampleTime=T
  Constant3 : Constant  Value=limit  SampleTime=T
  Delay : Delay  DelayLength=1  InitialCondition=0  SampleTime=T
  Delay1 : Delay  DelayLength=1  InitialCondition=0  SampleTime=T
  MATLAB Function : MATLAB Function  TreatAsAtomicUnit=on
  Rate Transition : RateTransition  OutPortSampleTime=T
  Out1 : Outport  VectorParamsAs1DForOutWhenUnconnected=off
  wires:
  MATLAB Function/2(uk) -> Out1/1
  MATLAB Function/1(temp) -> Delay1/1
  Constant1/1 -> MATLAB Function/4(Kp)
  Constant/1 -> MATLAB Function/6(T)
  Constant2/1 -> MATLAB Function/5(Ki)
  Delay/1 -> MATLAB Function/3(ek_1)
  Delay1/1 -> MATLAB Function/1(uk_1)
  Constant3/1 -> MATLAB Function/7(limit)
  In2/1 -> Rate Transition/1
  Rate Transition/1 -> MATLAB Function/2(ek), Delay/1

== system FOC_CHBI/CASECADED H-BRIDGE INVERTER/CONTROLLER/R_i1/iq ==
  In2 : Inport
  Constant : Constant  Value=T  SampleTime=T
  Constant1 : Constant  Value=Kp  SampleTime=T
  Constant2 : Constant  Value=Ki  SampleTime=T
  Constant3 : Constant  Value=limit  SampleTime=T
  Delay : Delay  DelayLength=1  InitialCondition=0  SampleTime=T
  Delay1 : Delay  DelayLength=1  InitialCondition=0  SampleTime=T
  MATLAB Function : MATLAB Function  TreatAsAtomicUnit=on
  Rate Transition : RateTransition  OutPortSampleTime=T
  Out1 : Outport  VectorParamsAs1DForOutWhenUnconnected=off
  wires:
  Rate Transition/1 -> Delay/1, MATLAB Function/2(ek)
  In2/1 -> Rate Transition/1
  Constant3/1 -> MATLAB Function/7(limit)
  Delay1/1 -> MATLAB Function/1(uk_1)
  Delay/1 -> MATLAB Function/3(ek_1)
  Constant2/1 -> MATLAB Function/5(Ki)
  Constant/1 -> MATLAB Function/6(T)
  Constant1/1 -> MATLAB Function/4(Kp)
  MATLAB Function/1(temp) -> Delay1/1
  MATLAB Function/2(uk) -> Out1/1

== system FOC_CHBI/CASECADED H-BRIDGE INVERTER/POWER CIRCUIT1/Subsystem/Subsystem1 ==
  PWM : Inport
  Breaker : spsBreakerLib/Breaker  InitialState=0  SwitchingTimes="[1/60  5/60]"  External=on  BreakerResistance=0.01  SnubberResistance=1e6  SnubberCapacitance=inf  Measurements=None  MoreParameters=on  NoBreakLoop=off
  Demux : Demux  Outputs=2
  IGBT/Diode{1..4} (4 alike) : spsIGBTDiodeLib/IGBT//Diode  Ron=1e-3  Rs=1e5  Cs=inf  Measurements=off
  Logical Operator : Logic  Operator=NOT  AllPortsSameDT=off  OutDataTypeStr=boolean
  Logical Operator1 : Logic  Operator=NOT  AllPortsSameDT=off  OutDataTypeStr=boolean
  Step : Step  Time=0  After=0  SampleTime=0
  A : PMIOPort  Side=Right
  B : PMIOPort  Port=2  Side=Right
  + : PMIOPort  Port=3  Side=Left
  - : PMIOPort  Port=4  Side=Left
  tag scope: eBH1=global
  wires:
  Step/1 -> Breaker/1, [eBH1]
  PWM/1 -> Demux/1
  Demux/1 -> IGBT/Diode1/1, Logical Operator/1
  Logical Operator/1 -> IGBT/Diode4/1
  Demux/2 -> IGBT/Diode3/1, Logical Operator1/1
  Logical Operator1/1 -> IGBT/Diode2/1
  connections:
  IGBT/Diode1/LConn1 -- +/RConn1 -- IGBT/Diode3/LConn1
  IGBT/Diode1/RConn1 -- A/RConn1 -- Breaker/LConn1 -- IGBT/Diode4/LConn1
  IGBT/Diode2/LConn1 -- B/RConn1 -- Breaker/RConn1 -- IGBT/Diode3/RConn1
  IGBT/Diode2/RConn1 -- -/RConn1 -- IGBT/Diode4/RConn1

== system FOC_CHBI/CASECADED H-BRIDGE INVERTER/POWER CIRCUIT1/Subsystem/Subsystem2 ==
  PWM : Inport
  Breaker : spsBreakerLib/Breaker  InitialState=0  SwitchingTimes="[1/60  5/60]"  External=on  BreakerResistance=0.01  SnubberResistance=1e6  SnubberCapacitance=inf  Measurements=None  MoreParameters=on  NoBreakLoop=off
  Demux : Demux  Outputs=2
  IGBT/Diode{1..4} (4 alike) : spsIGBTDiodeLib/IGBT//Diode  Ron=1e-3  Rs=1e5  Cs=inf  Measurements=off
  Logical Operator : Logic  Operator=NOT  AllPortsSameDT=off  OutDataTypeStr=boolean
  Logical Operator1 : Logic  Operator=NOT  AllPortsSameDT=off  OutDataTypeStr=boolean
  Step : Step  Time=0  After=0  SampleTime=0
  A : PMIOPort  Side=Right
  B : PMIOPort  Port=2  Side=Right
  + : PMIOPort  Port=3  Side=Left
  - : PMIOPort  Port=4  Side=Left
  tag scope: eBH2=global
  wires:
  Step/1 -> Breaker/1, [eBH2]
  Logical Operator1/1 -> IGBT/Diode2/1
  Demux/2 -> Logical Operator1/1, IGBT/Diode3/1
  Logical Operator/1 -> IGBT/Diode4/1
  Demux/1 -> Logical Operator/1, IGBT/Diode1/1
  PWM/1 -> Demux/1
  connections:
  IGBT/Diode4/RConn1 -- -/RConn1 -- IGBT/Diode2/RConn1
  IGBT/Diode3/RConn1 -- B/RConn1 -- Breaker/RConn1 -- IGBT/Diode2/LConn1
  IGBT/Diode4/LConn1 -- A/RConn1 -- Breaker/LConn1 -- IGBT/Diode1/RConn1
  IGBT/Diode3/LConn1 -- +/RConn1 -- IGBT/Diode1/LConn1

== system FOC_CHBI/CASECADED H-BRIDGE INVERTER/POWER CIRCUIT1/Subsystem/Subsystem3 ==
  PWM : Inport
  Breaker : spsBreakerLib/Breaker  InitialState=0  SwitchingTimes="[1/60  5/60]"  External=on  BreakerResistance=0.01  SnubberResistance=1e6  SnubberCapacitance=inf  Measurements=None  MoreParameters=on  NoBreakLoop=off
  Demux : Demux  Outputs=2
  IGBT/Diode{1..4} (4 alike) : spsIGBTDiodeLib/IGBT//Diode  Ron=1e-3  Rs=1e5  Cs=inf  Measurements=off
  Logical Operator : Logic  Operator=NOT  AllPortsSameDT=off  OutDataTypeStr=boolean
  Logical Operator1 : Logic  Operator=NOT  AllPortsSameDT=off  OutDataTypeStr=boolean
  Step : Step  Time=0  After=0  SampleTime=0
  A : PMIOPort  Side=Right
  B : PMIOPort  Port=2  Side=Right
  + : PMIOPort  Port=3  Side=Left
  - : PMIOPort  Port=4  Side=Left
  tag scope: eBH3=global
  wires:
  Step/1 -> Breaker/1, [eBH3]
  PWM/1 -> Demux/1
  Demux/1 -> IGBT/Diode1/1, Logical Operator/1
  Logical Operator/1 -> IGBT/Diode4/1
  Demux/2 -> IGBT/Diode3/1, Logical Operator1/1
  Logical Operator1/1 -> IGBT/Diode2/1
  connections:
  IGBT/Diode1/LConn1 -- +/RConn1 -- IGBT/Diode3/LConn1
  IGBT/Diode1/RConn1 -- A/RConn1 -- Breaker/LConn1 -- IGBT/Diode4/LConn1
  IGBT/Diode2/LConn1 -- B/RConn1 -- Breaker/RConn1 -- IGBT/Diode3/RConn1
  IGBT/Diode2/RConn1 -- -/RConn1 -- IGBT/Diode4/RConn1

== system FOC_CHBI/CASECADED H-BRIDGE INVERTER/POWER CIRCUIT1/Subsystem/Subsystem4 ==
  PWM : Inport
  Breaker : spsBreakerLib/Breaker  InitialState=0  SwitchingTimes="[1/60  5/60]"  External=on  BreakerResistance=0.01  SnubberResistance=1e6  SnubberCapacitance=inf  Measurements=None  MoreParameters=on  NoBreakLoop=off
  Demux : Demux  Outputs=2
  IGBT/Diode{1..4} (4 alike) : spsIGBTDiodeLib/IGBT//Diode  Ron=1e-3  Rs=1e5  Cs=inf  Measurements=off
  Logical Operator : Logic  Operator=NOT  AllPortsSameDT=off  OutDataTypeStr=boolean
  Logical Operator1 : Logic  Operator=NOT  AllPortsSameDT=off  OutDataTypeStr=boolean
  Step : Step  Time=0  After=0  SampleTime=0
  A : PMIOPort  Side=Right
  B : PMIOPort  Port=2  Side=Right
  + : PMIOPort  Port=3  Side=Left
  - : PMIOPort  Port=4  Side=Left
  tag scope: eBH4=global
  wires:
  Step/1 -> Breaker/1, [eBH4]
  Logical Operator1/1 -> IGBT/Diode2/1
  Demux/2 -> Logical Operator1/1, IGBT/Diode3/1
  Logical Operator/1 -> IGBT/Diode4/1
  Demux/1 -> Logical Operator/1, IGBT/Diode1/1
  PWM/1 -> Demux/1
  connections:
  IGBT/Diode4/RConn1 -- -/RConn1 -- IGBT/Diode2/RConn1
  IGBT/Diode3/RConn1 -- B/RConn1 -- Breaker/RConn1 -- IGBT/Diode2/LConn1
  IGBT/Diode4/LConn1 -- A/RConn1 -- Breaker/LConn1 -- IGBT/Diode1/RConn1
  IGBT/Diode3/LConn1 -- +/RConn1 -- IGBT/Diode1/LConn1

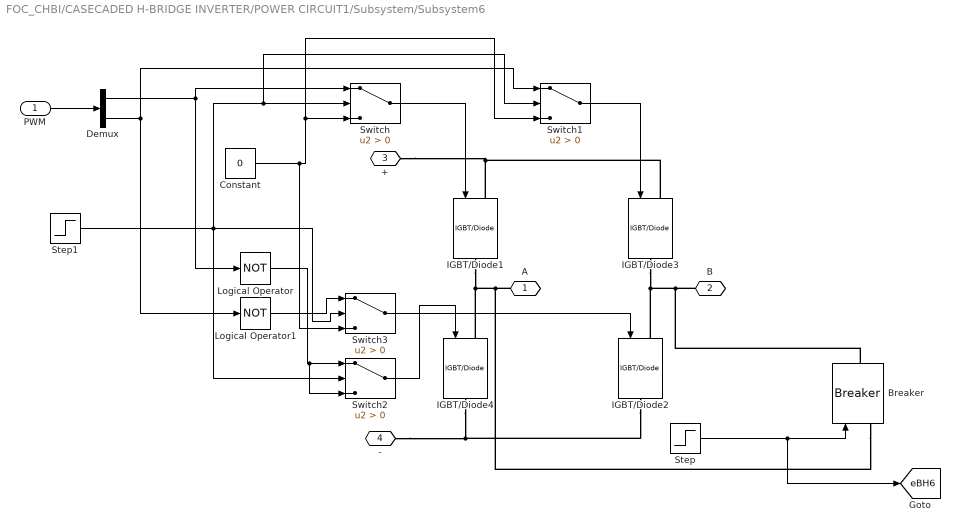
== system FOC_CHBI/CASECADED H-BRIDGE INVERTER/POWER CIRCUIT1/Subsystem/Subsystem6 ==
  PWM : Inport
  Breaker : spsBreakerLib/Breaker  InitialState=0  SwitchingTimes="[1/60  5/60]"  External=on  BreakerResistance=0.01  SnubberResistance=1e6  SnubberCapacitance=inf  Measurements=None  MoreParameters=on  NoBreakLoop=off
  Constant : Constant  Value=0
  Demux : Demux  Outputs=2
  IGBT/Diode{1..4} (4 alike) : spsIGBTDiodeLib/IGBT//Diode  Ron=1e-3  Rs=1e5  Cs=inf  Measurements=off
  Logical Operator : Logic  Operator=NOT  AllPortsSameDT=off  OutDataTypeStr=boolean
  Logical Operator1 : Logic  Operator=NOT  AllPortsSameDT=off  OutDataTypeStr=boolean
  Step : Step  Time=4  SampleTime=0
  Step1 : Step  Time=4  Before=1  After=-1  SampleTime=0
  Switch{,1..3} (4 alike) : Switch  Criteria=u2 > Threshold  SaturateOnIntegerOverflow=off  InputSameDT=off
  A : PMIOPort  Side=Right
  B : PMIOPort  Port=2  Side=Right
  + : PMIOPort  Port=3  Side=Left
  - : PMIOPort  Port=4  Side=Left
  tag scope: eBH6=global
  wires:
  Demux/2 -> Switch1/1, Logical Operator1/1
  Logical Operator/1 -> Switch2/3, Switch2/1
  Demux/1 -> Switch/1, Logical Operator/1
  PWM/1 -> Demux/1
  Step/1 -> [eBH6], Breaker/1
  Switch/1 -> IGBT/Diode1/1
  Switch1/1 -> IGBT/Diode3/1
  Switch2/1 -> IGBT/Diode4/1
  Logical Operator1/1 -> Switch3/1
  Switch3/1 -> IGBT/Diode2/1
  Constant/1 -> Switch/3, Switch1/3, Switch3/3
  Step1/1 -> Switch2/2, Switch3/2, Switch1/2, Switch/2
  connections:
  IGBT/Diode4/RConn1 -- -/RConn1 -- IGBT/Diode2/RConn1
  IGBT/Diode3/RConn1 -- Breaker/RConn1 -- B/RConn1 -- IGBT/Diode2/LConn1
  IGBT/Diode4/LConn1 -- Breaker/LConn1 -- A/RConn1 -- IGBT/Diode1/RConn1
  IGBT/Diode3/LConn1 -- +/RConn1 -- IGBT/Diode1/LConn1

== system FOC_CHBI/CASECADED H-BRIDGE INVERTER/POWER CIRCUIT1/Subsystem/Subsystem7 ==
  PWM : Inport
  Breaker : spsBreakerLib/Breaker  InitialState=0  SwitchingTimes="[1/60  5/60]"  External=on  BreakerResistance=0.01  SnubberResistance=1e6  SnubberCapacitance=inf  Measurements=None  MoreParameters=on  NoBreakLoop=off
  Constant : Constant  Value=0
  Demux : Demux  Outputs=2
  IGBT/Diode{1..4} (4 alike) : spsIGBTDiodeLib/IGBT//Diode  Ron=1e-3  Rs=1e5  Cs=inf  Measurements=off
  Logical Operator : Logic  Operator=NOT  AllPortsSameDT=off  OutDataTypeStr=boolean
  Logical Operator1 : Logic  Operator=NOT  AllPortsSameDT=off  OutDataTypeStr=boolean
  Step : Step  Time=4  SampleTime=0
  Step1 : Step  Time=4  Before=1  After=-1  SampleTime=0
  Switch{,1..3} (4 alike) : Switch  Criteria=u2 > Threshold  SaturateOnIntegerOverflow=off  InputSameDT=off
  A : PMIOPort  Side=Right
  B : PMIOPort  Port=2  Side=Right
  + : PMIOPort  Port=3  Side=Left
  - : PMIOPort  Port=4  Side=Left
  tag scope: eBH5=global
  wires:
  Demux/2 -> Switch1/1, Logical Operator1/1
  Logical Operator/1 -> Switch2/3, Switch2/1
  Demux/1 -> Switch/1, Logical Operator/1
  PWM/1 -> Demux/1
  Step/1 -> [eBH5], Breaker/1
  Switch/1 -> IGBT/Diode1/1
  Switch1/1 -> IGBT/Diode3/1
  Switch2/1 -> IGBT/Diode4/1
  Logical Operator1/1 -> Switch3/1
  Switch3/1 -> IGBT/Diode2/1
  Constant/1 -> Switch/3, Switch1/3, Switch3/3
  Step1/1 -> Switch2/2, Switch3/2, Switch1/2, Switch/2
  connections:
  IGBT/Diode4/RConn1 -- -/RConn1 -- IGBT/Diode2/RConn1
  IGBT/Diode3/RConn1 -- Breaker/RConn1 -- B/RConn1 -- IGBT/Diode2/LConn1
  IGBT/Diode4/LConn1 -- Breaker/LConn1 -- A/RConn1 -- IGBT/Diode1/RConn1
  IGBT/Diode3/LConn1 -- +/RConn1 -- IGBT/Diode1/LConn1

== system FOC_CHBI/CASECADED H-BRIDGE INVERTER/POWER CIRCUIT1/Subsystem1/Subsystem1 ==
  PWM : Inport
  Breaker : spsBreakerLib/Breaker  InitialState=0  SwitchingTimes="[1/60  5/60]"  External=on  BreakerResistance=0.01  SnubberResistance=1e6  SnubberCapacitance=inf  Measurements=None  MoreParameters=on  NoBreakLoop=off
  Demux : Demux  Outputs=2
  IGBT/Diode{1..4} (4 alike) : spsIGBTDiodeLib/IGBT//Diode  Ron=1e-3  Rs=1e5  Cs=inf  Measurements=off
  Logical Operator : Logic  Operator=NOT  AllPortsSameDT=off  OutDataTypeStr=boolean
  Logical Operator1 : Logic  Operator=NOT  AllPortsSameDT=off  OutDataTypeStr=boolean
  Step : Step  Time=0  After=0  SampleTime=0
  A : PMIOPort  Side=Right
  B : PMIOPort  Port=2  Side=Right
  + : PMIOPort  Port=3  Side=Left
  - : PMIOPort  Port=4  Side=Left
  tag scope: eCH1=global
  wires:
  Step/1 -> Breaker/1, [eCH1]
  PWM/1 -> Demux/1
  Demux/1 -> IGBT/Diode1/1, Logical Operator/1
  Logical Operator/1 -> IGBT/Diode4/1
  Demux/2 -> IGBT/Diode3/1, Logical Operator1/1
  Logical Operator1/1 -> IGBT/Diode2/1
  connections:
  IGBT/Diode1/LConn1 -- +/RConn1 -- IGBT/Diode3/LConn1
  IGBT/Diode1/RConn1 -- A/RConn1 -- Breaker/LConn1 -- IGBT/Diode4/LConn1
  IGBT/Diode2/LConn1 -- B/RConn1 -- Breaker/RConn1 -- IGBT/Diode3/RConn1
  IGBT/Diode2/RConn1 -- -/RConn1 -- IGBT/Diode4/RConn1

== system FOC_CHBI/CASECADED H-BRIDGE INVERTER/POWER CIRCUIT1/Subsystem1/Subsystem2 ==
  PWM : Inport
  Breaker : spsBreakerLib/Breaker  InitialState=0  SwitchingTimes="[1/60  5/60]"  External=on  BreakerResistance=0.01  SnubberResistance=1e6  SnubberCapacitance=inf  Measurements=None  MoreParameters=on  NoBreakLoop=off
  Demux : Demux  Outputs=2
  IGBT/Diode{1..4} (4 alike) : spsIGBTDiodeLib/IGBT//Diode  Ron=1e-3  Rs=1e5  Cs=inf  Measurements=off
  Logical Operator : Logic  Operator=NOT  AllPortsSameDT=off  OutDataTypeStr=boolean
  Logical Operator1 : Logic  Operator=NOT  AllPortsSameDT=off  OutDataTypeStr=boolean
  Step : Step  Time=0  After=0  SampleTime=0
  A : PMIOPort  Side=Right
  B : PMIOPort  Port=2  Side=Right
  + : PMIOPort  Port=3  Side=Left
  - : PMIOPort  Port=4  Side=Left
  tag scope: eCH2=global
  wires:
  Step/1 -> Breaker/1, [eCH2]
  Logical Operator1/1 -> IGBT/Diode2/1
  Demux/2 -> Logical Operator1/1, IGBT/Diode3/1
  Logical Operator/1 -> IGBT/Diode4/1
  Demux/1 -> Logical Operator/1, IGBT/Diode1/1
  PWM/1 -> Demux/1
  connections:
  IGBT/Diode4/RConn1 -- -/RConn1 -- IGBT/Diode2/RConn1
  IGBT/Diode3/RConn1 -- B/RConn1 -- Breaker/RConn1 -- IGBT/Diode2/LConn1
  IGBT/Diode4/LConn1 -- A/RConn1 -- Breaker/LConn1 -- IGBT/Diode1/RConn1
  IGBT/Diode3/LConn1 -- +/RConn1 -- IGBT/Diode1/LConn1

== system FOC_CHBI/CASECADED H-BRIDGE INVERTER/POWER CIRCUIT1/Subsystem1/Subsystem3 ==
  PWM : Inport
  Breaker : spsBreakerLib/Breaker  InitialState=0  SwitchingTimes="[1/60  5/60]"  External=on  BreakerResistance=0.01  SnubberResistance=1e6  SnubberCapacitance=inf  Measurements=None  MoreParameters=on  NoBreakLoop=off
  Demux : Demux  Outputs=2
  IGBT/Diode{1..4} (4 alike) : spsIGBTDiodeLib/IGBT//Diode  Ron=1e-3  Rs=1e5  Cs=inf  Measurements=off
  Logical Operator : Logic  Operator=NOT  AllPortsSameDT=off  OutDataTypeStr=boolean
  Logical Operator1 : Logic  Operator=NOT  AllPortsSameDT=off  OutDataTypeStr=boolean
  Step : Step  Time=0  After=0  SampleTime=0
  A : PMIOPort  Side=Right
  B : PMIOPort  Port=2  Side=Right
  + : PMIOPort  Port=3  Side=Left
  - : PMIOPort  Port=4  Side=Left
  tag scope: eCH3=global
  wires:
  Step/1 -> Breaker/1, [eCH3]
  PWM/1 -> Demux/1
  Demux/1 -> IGBT/Diode1/1, Logical Operator/1
  Logical Operator/1 -> IGBT/Diode4/1
  Demux/2 -> IGBT/Diode3/1, Logical Operator1/1
  Logical Operator1/1 -> IGBT/Diode2/1
  connections:
  IGBT/Diode1/LConn1 -- +/RConn1 -- IGBT/Diode3/LConn1
  IGBT/Diode1/RConn1 -- A/RConn1 -- Breaker/LConn1 -- IGBT/Diode4/LConn1
  IGBT/Diode2/LConn1 -- B/RConn1 -- Breaker/RConn1 -- IGBT/Diode3/RConn1
  IGBT/Diode2/RConn1 -- -/RConn1 -- IGBT/Diode4/RConn1
